simulink model "Control_Loop"  (R2016a)
settings: Solver=FixedStepAuto  StartTime=0.0  StopTime=50  FixedStep=.0001  RelTol=1e-3
settings Model: Creator=Jet  LastModifiedBy=Jet

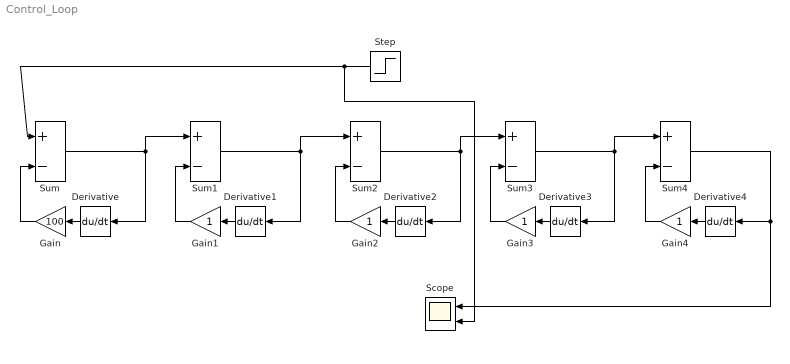
== system Control_Loop ==
  Derivative{,1..4} (5 alike) : Derivative
  Gain : Gain  Gain=100
  Gain{1..4} (4 alike) : Gain
  Scope : Scope  NumInputPorts=2
  Step : Step  SampleTime=0
  Sum{,1..4} (5 alike) : Sum  Inputs=+-
  wires:
  Sum/1 -> Sum1/1, Derivative/1
  Sum2/1 -> Sum3/1, Derivative2/1
  Sum4/1 -> Scope/1, Derivative4/1
  Derivative/1 -> Gain/1
  Gain/1 -> Sum/2
  Sum1/1 -> Derivative1/1, Sum2/1
  Derivative1/1 -> Gain1/1
  Gain1/1 -> Sum1/2
  Derivative2/1 -> Gain2/1
  Gain2/1 -> Sum2/2
  Sum3/1 -> Derivative3/1, Sum4/1
  Derivative3/1 -> Gain3/1
  Gain3/1 -> Sum3/2
  Derivative4/1 -> Gain4/1
  Gain4/1 -> Sum4/2
  Step/1 -> Sum/1, Scope/2
